simulink model "second_order_sim"  (R2023a)
settings: Solver=VariableStepAuto  StartTime=0.0  StopTime=0.03  RelTol=1e-3
values from neighbouring files (symbols this model uses):
  omega = 2 .* pi .* freq    [second_order_code.m]
  t_step = 1e-6    (= 1e-06)    [second_order_code.m]
settings Model: Creator=McAtr1Xx  LastModifiedBy=McAtr1Xx

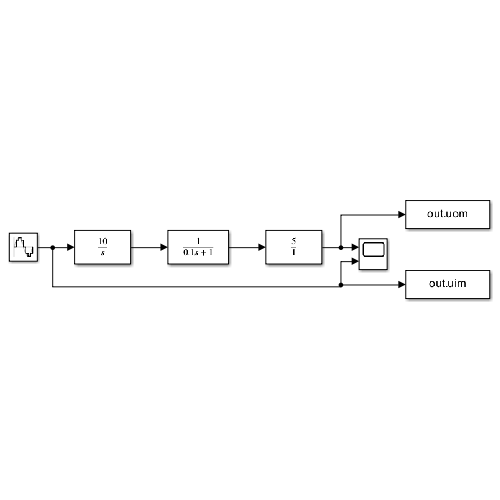
[thumbnail: Simulink's stored preview of the top-level diagram]
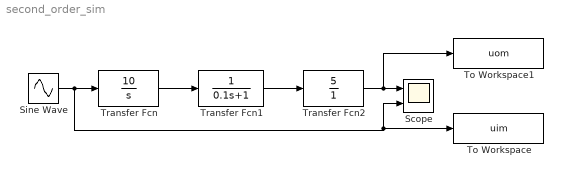
== system second_order_sim ==
  Scope : Scope  NumInputPorts=2
  Sine Wave : Sin  Frequency=omega  SampleTime=t_step
  To Workspace : ToWorkspace  VariableName=uim  SaveFormat=Timeseries  SampleTime=-1
  To Workspace1 : ToWorkspace  VariableName=uom  SaveFormat=Timeseries  SampleTime=-1
  Transfer Fcn : TransferFcn  Numerator=[10]  Denominator=[1 0]
  Transfer Fcn1 : TransferFcn  Denominator=[0.1 1]
  Transfer Fcn2 : TransferFcn  Numerator=[5]  Denominator=[1]
  wires:
  Transfer Fcn2/1 -> To Workspace1/1, Scope/1
  Transfer Fcn1/1 -> Transfer Fcn2/1
  Transfer Fcn/1 -> Transfer Fcn1/1
  Sine Wave/1 -> Scope/2, To Workspace/1, Transfer Fcn/1
